simulink model "VB_RIFKF_UWB_INS25"  (R2023a)
settings: Solver=FixedStepAuto  StartTime=0.0  StopTime=500  FixedStep=0.01  RelTol=1e-3
InitFcn:
  | resilient_initNavigation1216;
  | init_param;
  | param_bias;
undefined symbols (not defined in the file or in its folder): dt, g0, gam0_rad, ISUS_flag, lp_GPS_sample_time, lp_Lidar_knoise, lp_Lidar_max, lp_Lidar_min, lp_Lidar_sample_time, lp_Lidar_seed, lp_UWB_knoise, lp_UWB_sample_time, lp_UWB_seed, lp_UWB_XY_max, lp_UWB_XY_min, magnitude, p, P0, P0_RIEKF, param, pd0, pe0, phi0_rad, pn0, psi, psi0_rad, state_dim, vd0, ve0, vn0
libraries: simulink_extras x108, simulink x89, dspstat3 x74, sharedtransform x61, matrix_library x11, sharedTrackingLibrary x8, aerolibconvert2 x5, aerolibtransform2 x5, dspfactors x3
(part 15 of 29)

== system VB_RIFKF_UWB_INS25/ISUS_RIEKF3/INS propogation3/att update ==
  dtheta : Inport
  gyro : Inport  Port=2
  quat_0 : Inport  Port=3  PortDimensions=4
  init_flag : Inport  Port=4
  Bus Creator1 : BusCreator  Inputs=1
  Constant : Constant  Value=dt
  Delay1 : Delay  DelayLength=1  InitialConditionSource=Input port  InitialCondition=0  ExternalReset=Level hold
      settings: InputPortMap=u0,r5,p4
  Detect Increase : simulink/Logic and Bit Operations/Detect Increase  vinit=0.0  OutDataTypeStr=boolean
  MATLAB Function : MATLAB Function  TreatAsAtomicUnit=on
  MATLAB Function2 : MATLAB Function  TreatAsAtomicUnit=on
  Quaternions to Direction Cosine Matrix : sharedtransform/Quaternions to  Direction Cosine Matrix  aMode=aMode
      settings: LibrarySourceBlock=|
      | aerolibtransform2/Quaternions to
      | Direction Cosine Matrix
  Scope : Scope
  Transpose : Math  Operator=transpose
  att_update1 : Outport
  wires:
  init_flag/1 -> Detect Increase/1
  quat_0/1 -> Quaternions to Direction Cosine Matrix/1
  gyro/1 -> MATLAB Function/2(w)  "w"
  Constant/1 -> MATLAB Function/3(dt)
  Quaternions to Direction Cosine Matrix/1 -> Transpose/1
  Transpose/1 -> Delay1/3
  Delay1/1 -> MATLAB Function/1(Rbn_k_1)
  Detect Increase/1 -> Delay1/2
  Bus Creator1/1 -> Delay1/1, att_update1/1
  MATLAB Function/1(Rbn) -> MATLAB Function2/2(Rbn)  "DCM_b_n"
  MATLAB Function2/1(Rbn_correct) -> Bus Creator1/1  "DCM_b_n"
  dtheta/1 -> MATLAB Function2/1(delta), Scope/1

== system VB_RIFKF_UWB_INS25/ISUS_RIEKF3/INS propogation3/gyro bias compensation ==
  raw <gyro_B_rad/s_LPF> : Inport
  ddg : Inport  Port=2
  Measuemrnt Enable Flag : Inport  Port=3
  QGC_init : Inport  Port=4
  Add1 : Sum
  Data Type Conversion4 : DataTypeConversion  OutDataTypeStr=single  SaturateOnIntegerOverflow=off  RndMeth=Floor
  Scope1 : Scope
  error compensation : Subsystem
      settings: PortSchema="{\"entries\":[{\"content\":{\"sides\":[{\"content\":{\"connectorIds\":[\"In1\",\"In2\"]},\"type\":\"ConnectorPlacement.EquallySpacedRectSide\",\"uuid\":\"380e61a1-8124-48da-8c16-e78a4b6c30a9\"},{\"content\":{\"connectorIds\":[\"Out1\"],\"side\":\"RIGHT\"},\"type\":\"ConnectorPlacement.EquallySpacedRectSide\",\"uuid\":\"dacfd24e-67c3-4852-b5f7-795187362148\"},{\"content\":{\"side\":\"TOP\"},\"type\":\"ConnectorPlacement.EquallySpacedRectSide\",\"uuid\":\"56579dc4-3963-4476-a5d7-e0c30cfcd11c\"},{\"content\":{\"connectorIds\":[\"In3\"],\"side\":\"BOTTOM\"},\"type\":\"ConnectorPlacement.EquallySpacedRectSide\",\"uuid\":\"fc24e139-e918-40f2-99cc-0ca16c0a4a58\"}]},\"type\":\"ConnectorPlacement.EquallySpacedConnector\",\"uuid\":\"3ce5c04a-f8d2-476b-8ef1-0541292dfd95\"}],\"packageUris\":[\"http://schema.mathworks.com/mf0/Connector/R2020b\"],\"version\":\"1.0\"}"
  wb : Outport  PortDimensions=3
  dg : Outport  Port=2  PortDimensions=3
  wires:
  Data Type Conversion4/1 -> wb/1
  raw <gyro_B_rad/s_LPF>/1 -> Add1/1
  error compensation/1(dg) -> Add1/2, Scope1/1, dg/1
  Measuemrnt Enable Flag/1 -> error compensation/2(Enable)
  Add1/1 -> Data Type Conversion4/1
  QGC_init/1 -> error compensation/3(QGC_init)
  ddg/1 -> error compensation/1(ddg)

== system VB_RIFKF_UWB_INS25/ISUS_RIEKF3/INS propogation3/vel//pos update ==
  dtheta : Inport
  <DCM_b_n> : Inport  Port=2
  Ab : Inport  Port=3
  v0 : Inport  Port=4
  p0 : Inport  Port=5
  QGC_init : Inport  Port=6
  dp : Inport  Port=7
  dv : Inport  Port=8
  Kinematic Equation : Subsystem
  QGC_init1 : InportShadow  Port=6
  pos update : Subsystem
  vel update : Subsystem
  p_k : Outport  PortDimensions=3
  V : Outport  Port=2  PortDimensions=3
  wires:
  QGC_init1/1 -> pos update/4(QGC_init)
  pos update/1(p_k) -> p_k/1
  p0/1 -> pos update/5(p0)
  dp/1 -> pos update/3(dp)
  v0/1 -> vel update/5(v0)
  dv/1 -> vel update/4(KFState_dv)
  Kinematic Equation/1(An) -> vel update/3(An)
  QGC_init/1 -> vel update/2(QGC_init)
  Ab/1 -> Kinematic Equation/2(Ab)
  <DCM_b_n>/1 -> Kinematic Equation/1(Cbn)
  vel update/1(vel_k) -> V/1, pos update/2(vel_k)
  dtheta/1 -> pos update/1(dtheta), vel update/1(dtheta)

== system VB_RIFKF_UWB_INS25/ISUS_RIEKF3/Subsystem/ISIU ==
  xk_k_1 : Inport
  xk_k_2 : Inport  Port=2
  xk_k_3 : Inport  Port=3
  pk_k_1 : Inport  Port=4
  pk_k_2 : Inport  Port=5
  pk_k_3 : Inport  Port=6
  1222bk : MATLAB Function  Commented=on  TreatAsAtomicUnit=on
  1222bk02 : MATLAB Function  Commented=on  TreatAsAtomicUnit=on
  Constant : Constant  Value=3
  Constant1 : Constant  OutDataTypeStr=boolean
  Constant11 : Constant  Commented=on  Value=[0.9;0.05;0.05]  OutDataTypeStr=single
  Data Type Conversion : DataTypeConversion  OutDataTypeStr=single  SaturateOnIntegerOverflow=off  RndMeth=Floor
  Data Type Conversion1 : DataTypeConversion  Commented=on  OutDataTypeStr=single  SaturateOnIntegerOverflow=off  RndMeth=Floor
  Delay1 : Delay  Commented=on  DelayLength=1  InitialConditionSource=Input port
      settings: InputPortMap=u0,p4
  Delay4 : Delay  Commented=on  DelayLength=1  InitialConditionSource=Input port
      settings: InputPortMap=u0,p4
  Digital Clock1 : DigitalClock  SampleTime=0.01
  MATLAB Function : MATLAB Function  TreatAsAtomicUnit=on
  MATLAB Function3 : MATLAB Function  Commented=on  TreatAsAtomicUnit=on
  MATLAB Function4 : MATLAB Function  TreatAsAtomicUnit=on
  Scope : Scope
  xk_k : Outport
  pk_k : Outport  Port=2
  xk_k_o1 : Outport  Port=3
  xk_k_o2 : Outport  Port=4
  xk_k_o3 : Outport  Port=5
  pk_k_o1 : Outport  Port=6
  pk_k_o2 : Outport  Port=7
  pk_k_o3 : Outport  Port=8
  wires:
  MATLAB Function/8(P_cov_system) -> pk_k/1
  MATLAB Function/7(system_pos) -> xk_k/1
  MATLAB Function/6(object3_cov) -> pk_k_o3/1
  MATLAB Function/5(object3_pos) -> xk_k_o3/1
  MATLAB Function/4(object2_cov) -> pk_k_o2/1
  MATLAB Function/3(object2_pos) -> xk_k_o2/1
  MATLAB Function/2(object1_cov) -> pk_k_o1/1
  MATLAB Function/1(object1_pos) -> xk_k_o1/1
  Data Type Conversion/1 -> Delay4/1
  Constant11/1 -> Delay4/2
  Data Type Conversion1/1 -> Delay1/1
  Constant/1 -> MATLAB Function/9(N)
  xk_k_3/1 -> MATLAB Function/8(object3_correct_pos)
  xk_k_2/1 -> MATLAB Function/7(object2_correct_pos)
  xk_k_1/1 -> MATLAB Function/6(object1_correct_pos)
  pk_k_3/1 -> MATLAB Function/3(inform_object3_correct)
  pk_k_2/1 -> MATLAB Function/2(inform_object2_correct)
  pk_k_1/1 -> MATLAB Function/1(inform_object1_correct)
  Constant1/1 -> MATLAB Function/10(flag), MATLAB Function4/2(u)
  Digital Clock1/1 -> MATLAB Function4/1(t)

== system VB_RIFKF_UWB_INS25/ISUS_RIEKF3/Subsystem/Subsystem ==
  X_mixed_RIEKF_M1 : Inport
  Bus Creator : BusCreator  Inputs=5
  Bus Creator1 : BusCreator  Inputs=1
  Selector : Selector  InputPortWidth=15  IndexOptions=Index vector (dialog)  Indices=[1 2 3]  OutputSizes=1
  Selector1 : Selector  InputPortWidth=15  IndexOptions=Index vector (dialog)  Indices=[4 5 6]  OutputSizes=1
  Selector2 : Selector  InputPortWidth=15  IndexOptions=Index vector (dialog)  Indices=[7 8 9]  OutputSizes=1
  Selector3 : Selector  InputPortWidth=15  IndexOptions=Index vector (dialog)  Indices=[10 11 12]  OutputSizes=1
  Selector4 : Selector  InputPortWidth=15  IndexOptions=Index vector (dialog)  Indices=[13 14 15]  OutputSizes=1
  Out1 : Outport
  wires:
  Selector3/1 -> Bus Creator/4  "KFState_dg"
  Selector1/1 -> Bus Creator/2  "KFState_dv"
  Selector2/1 -> Bus Creator/3  "KFState_dp"
  Bus Creator/1 -> Bus Creator1/1  "delta_state"
  Selector4/1 -> Bus Creator/5  "KFState_da"
  X_mixed_RIEKF_M1/1 -> Selector4/1, Selector3/1, Selector2/1, Selector1/1, Selector/1
  Selector/1 -> Bus Creator/1  "KFState_dtheta"
  Bus Creator1/1 -> Out1/1

== system VB_RIFKF_UWB_INS25/ISUS_RIEKF3/Subsystem/Subsystem1 ==
  X_mixed_RIEKF_M1 : Inport
  Bus Creator : BusCreator  Inputs=5
  Bus Creator1 : BusCreator  Inputs=1
  Selector : Selector  InputPortWidth=15  IndexOptions=Index vector (dialog)  Indices=[1 2 3]  OutputSizes=1
  Selector1 : Selector  InputPortWidth=15  IndexOptions=Index vector (dialog)  Indices=[4 5 6]  OutputSizes=1
  Selector2 : Selector  InputPortWidth=15  IndexOptions=Index vector (dialog)  Indices=[7 8 9]  OutputSizes=1
  Selector3 : Selector  InputPortWidth=15  IndexOptions=Index vector (dialog)  Indices=[10 11 12]  OutputSizes=1
  Selector4 : Selector  InputPortWidth=15  IndexOptions=Index vector (dialog)  Indices=[13 14 15]  OutputSizes=1
  Out1 : Outport
  wires:
  Bus Creator1/1 -> Out1/1
  Selector/1 -> Bus Creator/1  "KFState_dtheta"
  X_mixed_RIEKF_M1/1 -> Selector/1, Selector1/1, Selector2/1, Selector3/1, Selector4/1
  Selector4/1 -> Bus Creator/5  "KFState_da"
  Bus Creator/1 -> Bus Creator1/1  "delta_state"
  Selector2/1 -> Bus Creator/3  "KFState_dp"
  Selector1/1 -> Bus Creator/2  "KFState_dv"
  Selector3/1 -> Bus Creator/4  "KFState_dg"

== system VB_RIFKF_UWB_INS25/ISUS_RIEKF3/Subsystem/Subsystem2 ==
  X_mixed_RIEKF_M1 : Inport
  Bus Creator : BusCreator  Inputs=5
  Bus Creator1 : BusCreator  Inputs=1
  Selector : Selector  InputPortWidth=15  IndexOptions=Index vector (dialog)  Indices=[1 2 3]  OutputSizes=1
  Selector1 : Selector  InputPortWidth=15  IndexOptions=Index vector (dialog)  Indices=[4 5 6]  OutputSizes=1
  Selector2 : Selector  InputPortWidth=15  IndexOptions=Index vector (dialog)  Indices=[7 8 9]  OutputSizes=1
  Selector3 : Selector  InputPortWidth=15  IndexOptions=Index vector (dialog)  Indices=[10 11 12]  OutputSizes=1
  Selector4 : Selector  InputPortWidth=15  IndexOptions=Index vector (dialog)  Indices=[13 14 15]  OutputSizes=1
  Out1 : Outport
  wires:
  Selector3/1 -> Bus Creator/4  "KFState_dg"
  Selector1/1 -> Bus Creator/2  "KFState_dv"
  Selector2/1 -> Bus Creator/3  "KFState_dp"
  Bus Creator/1 -> Bus Creator1/1  "delta_state"
  Selector4/1 -> Bus Creator/5  "KFState_da"
  X_mixed_RIEKF_M1/1 -> Selector4/1, Selector3/1, Selector2/1, Selector1/1, Selector/1
  Selector/1 -> Bus Creator/1  "KFState_dtheta"
  Bus Creator1/1 -> Out1/1

== system VB_RIFKF_UWB_INS25/ISUS_RIEKF3/Subsystem/Subsystem3 ==
  X_mixed_RIEKF_M1 : Inport
  Bus Creator : BusCreator  Inputs=5
  Bus Creator1 : BusCreator  Inputs=1
  Selector : Selector  InputPortWidth=15  IndexOptions=Index vector (dialog)  Indices=[1 2 3]  OutputSizes=1
  Selector1 : Selector  InputPortWidth=15  IndexOptions=Index vector (dialog)  Indices=[4 5 6]  OutputSizes=1
  Selector2 : Selector  InputPortWidth=15  IndexOptions=Index vector (dialog)  Indices=[7 8 9]  OutputSizes=1
  Selector3 : Selector  InputPortWidth=15  IndexOptions=Index vector (dialog)  Indices=[10 11 12]  OutputSizes=1
  Selector4 : Selector  InputPortWidth=15  IndexOptions=Index vector (dialog)  Indices=[13 14 15]  OutputSizes=1
  Out1 : Outport
  wires:
  Bus Creator1/1 -> Out1/1
  Selector/1 -> Bus Creator/1  "KFState_dtheta"
  X_mixed_RIEKF_M1/1 -> Selector/1, Selector1/1, Selector2/1, Selector3/1, Selector4/1
  Selector4/1 -> Bus Creator/5  "KFState_da"
  Bus Creator/1 -> Bus Creator1/1  "delta_state"
  Selector2/1 -> Bus Creator/3  "KFState_dp"
  Selector1/1 -> Bus Creator/2  "KFState_dv"
  Selector3/1 -> Bus Creator/4  "KFState_dg"

== system VB_RIFKF_UWB_INS25/No.1_Sensor_Data_Process/GPS_Data_Process/LLA2NED ==
  note: Vecef2ned
  gps_LLA_rad : Inport
  GPSfixtype : Inport  Port=2
  GPS_Vecef_m/s : Inport  Port=3
  QGC_sensor_reinit : Inport  Port=4
  Angle Conversion1 : aerolibconvert2/Angle Conversion  IU=deg  OU=rad
  Bus Creator : BusCreator  Inputs=3
  Bus Creator1 : BusCreator  Inputs=3
  Bus Creator2 : BusCreator  Inputs=3
  Bus Selector : BusSelector  OutputSignals=lon_gps,lat_gps
  Bus Selector1 : BusSelector  OutputSignals=lat_gps,lon_gps,H_gps
  Constant1 : Constant  Value=-90
  Constant4 : Constant  Value=0
  Data Type Conversion{,1..6} (7 alike) : DataTypeConversion  OutDataTypeStr=single  SaturateOnIntegerOverflow=off  RndMeth=Floor
  Demux{,1..3} (4 alike) : Demux  Outputs=3
  Detect Increase : simulink/Logic and Bit Operations/Detect Increase  vinit=0.0  OutDataTypeStr=boolean
  Digital Clock : DigitalClock  SampleTime=0.01
  Direction Cosine Matrix ECEF to NED : aerolibtransform2/Direction Cosine Matrix ECEF to NED  Commented=on
  Divide1 : Product  Inputs=**  Multiplication=Matrix(*)
  Gain : Gain  Gain=-1
  LLA to ECEF Position : LLA2ECEF  R=6378137
  LLA to ECEF Position1 : LLA2ECEF  R=6378137
  MATLAB Function2 : MATLAB Function  TreatAsAtomicUnit=on
  Mux2 : Mux  Inputs=3
  Mux5 : Mux  Inputs=2
  Mux6 : Mux  Inputs=2
  Product : Product  Commented=on  Multiplication=Matrix(*)
  Radians to Degrees{,1..3} (4 alike) : simulink_extras/Transformations/Radians to Degrees
  Radians to Degrees4 : simulink_extras/Transformations/Radians to Degrees  Commented=on
  Rotation Angles to Direction Cosine Matrix : sharedtransform/Rotation Angles to Direction Cosine Matrix  rotationOrder=ZYX  aMode=aMode
  Scope : Scope  NumInputPorts=2
  Scope1 : Scope
  Scope2 : Scope  NumInputPorts=2
  Selector2 : Selector  Commented=on  InputPortWidth=3  IndexOptions=Index vector (dialog)  Indices=[1 2]  OutputSizes=1
  Sum : Sum  Inputs=|++
  Sum1 : Sum  Inputs=|+-
  initGPSLLA : MATLAB Function  TreatAsAtomicUnit=on
  "gpsposNEDout " : Outport
  gpsvNEDout : Outport  Port=2
  GPS0 : Outport  Port=3
  gpsposNED_noerr : Outport  Port=4
  wires:
  initGPSLLA/2(init_GPSLLAflag) -> Scope/1
  initGPSLLA/1(gpsLLA0_rad) -> Scope/2, Demux/1
  Detect Increase/1 -> initGPSLLA/1(QGCinitflag)
  Data Type Conversion3/1 -> gpsvNEDout/1  "gpspos_N"
  Radians to Degrees4/1 -> Direction Cosine Matrix ECEF to NED/1
  Selector2/1 -> Radians to Degrees4/1
  Direction Cosine Matrix ECEF to NED/1 -> Product/1
  GPS_Vecef_m/s/1 -> Product/2, Data Type Conversion3/1
  Radians to Degrees3/1 -> Mux5/2
  Radians to Degrees2/1 -> Mux5/1
  Angle Conversion1/1 -> Sum/2
  Data Type Conversion2/1 -> Bus Creator1/3  "gpspos_D"
  Data Type Conversion1/1 -> Bus Creator1/2  "gpspos_E"
  Data Type Conversion/1 -> Bus Creator1/1  "gpspos_N"
  QGC_sensor_reinit/1 -> Detect Increase/1
  Radians to Degrees1/1 -> Mux6/2
  Radians to Degrees/1 -> Mux6/1
  gps_LLA_rad/1 -> Demux1/1, Selector2/1, initGPSLLA/3(gps_LLA_rad)
  Bus Selector1/3 -> LLA to ECEF Position/2  "<H_gps>"
  Bus Selector1/2 -> Radians to Degrees3/1  "<lon_gps>"
  Bus Selector1/1 -> Radians to Degrees2/1  "<lat_gps>"
  Bus Selector/1 -> Mux2/1  "<lon_gps>"
  Bus Selector/2 -> Gain/1  "<lat_gps>"
  Sum/1 -> Mux2/2
  Demux1/2 -> Radians to Degrees1/1
  LLA to ECEF Position/1 -> Sum1/2
  Constant1/1 -> Angle Conversion1/1
  Rotation Angles to Direction Cosine Matrix/1 -> Divide1/1
  Mux2/1 -> Rotation Angles to Direction Cosine Matrix/1
  Demux1/1 -> Radians to Degrees/1
  Sum1/1 -> Divide1/2
  Constant4/1 -> Mux2/3
  LLA to ECEF Position1/1 -> Sum1/1
  Gain/1 -> Sum/1
  Mux5/1 -> LLA to ECEF Position/1
  Mux6/1 -> LLA to ECEF Position1/1
  Demux1/3 -> LLA to ECEF Position1/2
  Demux/1 -> Bus Creator/1  "lat_gps"
  Demux/2 -> Bus Creator/2  "lon_gps"
  Demux/3 -> Bus Creator/3  "H_gps"
  Bus Creator/1 -> GPS0/1, Bus Selector1/1, Bus Selector/1
  Demux3/1 -> Data Type Conversion/1  "gpspos_N"
  Demux3/2 -> Data Type Conversion1/1  "gpspos_E"
  Demux3/3 -> Data Type Conversion2/1  "gpspos_D"
  Bus Creator1/1 -> Scope1/1, "gpsposNEDout "/1
  GPSfixtype/1 -> initGPSLLA/2(GPSfixtype)
  Digital Clock/1 -> MATLAB Function2/1(t)
  Bus Creator2/1 -> gpsposNED_noerr/1
  Demux2/3 -> Data Type Conversion6/1  "gpspos_D"
  Demux2/2 -> Data Type Conversion5/1  "gpspos_E"
  Demux2/1 -> Data Type Conversion4/1  "gpspos_N"
  Data Type Conversion4/1 -> Bus Creator2/1  "gpspos_N"
  Data Type Conversion5/1 -> Bus Creator2/2  "gpspos_E"
  Data Type Conversion6/1 -> Bus Creator2/3  "gpspos_D"
  Divide1/1 -> Demux3/1, Scope2/1, Demux2/1, Scope2/2, MATLAB Function2/2(u)

== system VB_RIFKF_UWB_INS25/No.1_Sensor_Data_Process/GPS_Data_Process/heading_GPS ==
  Vned : Inport
  Atan2 : Trigonometry  Operator=atan2
  Compare To Constant : simulink/Logic and Bit Operations/Compare To Constant  relop=>=  const=0.8  OutDataTypeStr=boolean
  Math Function : Math  Operator=magnitude^2  SignedPower=on
  Moving Average1 : dspstat3/Moving Average  Commented=on  Method=Sliding window  ForgettingFactorPort=off  SpecifyWindowLength=on  WindowLength=10  OverlapLength=9  AllowArbitraryInputLength=off  ForgettingFactor=0.9  SimulateUsing=Code generation
  Scope : Scope  NumInputPorts=2
  Scope1 : Scope
  Selector2 : Selector  InputPortWidth=3  IndexOptions=Index vector (dialog)  Indices=[2]  OutputSizes=1
  Selector3 : Selector  InputPortWidth=3  IndexOptions=Index vector (dialog)  Indices=[1]  OutputSizes=1
  Selector4 : Selector  InputPortWidth=3  IndexOptions=Index vector (dialog)  Indices=[1 2]  OutputSizes=1
  Sqrt : Sqrt
  Sum of Elements : Sum  Inputs=+
  heading_GPS_rad : Outport
  heading_GPS_valid : Outport  Port=2
  wires:
  Atan2/1 -> heading_GPS_rad/1, Scope/2, Scope/1
  Compare To Constant/1 -> heading_GPS_valid/1, Scope1/1
  Sqrt/1 -> Compare To Constant/1
  Selector4/1 -> Math Function/1
  Sum of Elements/1 -> Sqrt/1
  Selector3/1 -> Atan2/2
  Vned/1 -> Selector3/1, Selector4/1, Selector2/1
  Math Function/1 -> Sum of Elements/1
  Selector2/1 -> Atan2/1

== system VB_RIFKF_UWB_INS25/No.1_Sensor_Data_Process/IMU_Data_Process/Bias Eliminate ==
  gyro_B_rad/s_ori : Inport
  Data Type Conversion : DataTypeConversion  OutDataTypeStr=single  SaturateOnIntegerOverflow=off  RndMeth=Floor
  Digital Clock : DigitalClock
  Memory : Memory
  Scope : Scope
  Subsystem : Subsystem
  Sum : Sum  Inputs=|+-
  Switch : Switch  Criteria=u2 > Threshold  Threshold=5  SaturateOnIntegerOverflow=off  InputSameDT=off
  Out1 : Outport
  wires:
  Memory/1 -> Switch/1
  Switch/1 -> Memory/1, Scope/1
  Subsystem/1(mean_data) -> Switch/3
  Digital Clock/1 -> Switch/2
  Sum/1 -> Data Type Conversion/1
  gyro_B_rad/s_ori/1 -> Sum/1, Subsystem/1(data)
  Data Type Conversion/1 -> Out1/1

== system VB_RIFKF_UWB_INS25/No.1_Sensor_Data_Process/IMU_Data_Process/accl_preprocessing2 ==
  note: front-right-dowm
  accl_B_m/s_ori : Inport
  Constant2 : Constant  Value=1/dt  OutDataTypeStr=single
  Constant4 : Constant  Value=1/dt  OutDataTypeStr=single
  Constant6 : Constant  Value=1/dt  OutDataTypeStr=single
  Constant7 : Constant  Value=param.proces.imu_gyro_cutoff_freq  OutDataTypeStr=single
  Demux : Demux  Outputs=3
  MATLAB Function1 : MATLAB Function  TreatAsAtomicUnit=on
  MATLAB Function2 : MATLAB Function  TreatAsAtomicUnit=on
  MATLAB Function3 : MATLAB Function  TreatAsAtomicUnit=on
  Vector Concatenate : Concatenate  NumInputs=3
  accl_B_m/s2_LPF : Outport
  wires:
  MATLAB Function2/1(curr_output) -> Vector Concatenate/1  "wx"
  MATLAB Function1/1(curr_output) -> Vector Concatenate/2  "wy"
  MATLAB Function3/1(curr_output) -> Vector Concatenate/3  "wz"
  Constant7/1 -> MATLAB Function1/3(cutoff_freq), MATLAB Function3/3(cutoff_freq), MATLAB Function2/3(cutoff_freq)
  Demux/3 -> MATLAB Function3/1(curr_input)
  Constant6/1 -> MATLAB Function3/2(sample_freq)
  Demux/2 -> MATLAB Function1/1(curr_input)
  Demux/1 -> MATLAB Function2/1(curr_input)
  accl_B_m/s_ori/1 -> Demux/1
  Constant2/1 -> MATLAB Function1/2(sample_freq)
  Constant4/1 -> MATLAB Function2/2(sample_freq)
  Vector Concatenate/1 -> accl_B_m/s2_LPF/1

== system VB_RIFKF_UWB_INS25/No.1_Sensor_Data_Process/IMU_Data_Process/gyro_preprocessing2 ==
  note: rad/s
  note: front-right-dowm
  gyro_B_rad/s_ori : Inport
  Constant2 : Constant  Value=1/dt  OutDataTypeStr=single
  Constant4 : Constant  Value=1/dt  OutDataTypeStr=single
  Constant6 : Constant  Value=1/dt  OutDataTypeStr=single
  Constant7 : Constant  Value=param.proces.imu_gyro_cutoff_freq  OutDataTypeStr=single
  Demux : Demux  Outputs=3
  MATLAB Function1 : MATLAB Function  TreatAsAtomicUnit=on
  MATLAB Function2 : MATLAB Function  TreatAsAtomicUnit=on
  MATLAB Function3 : MATLAB Function  TreatAsAtomicUnit=on
  Scope : Scope  NumInputPorts=2
  Vector Concatenate : Concatenate  NumInputs=3
  gyro_B_rad/s_LPF : Outport  PortDimensions=3
  wires:
  Vector Concatenate/1 -> gyro_B_rad/s_LPF/1
  Constant4/1 -> MATLAB Function2/2(sample_freq)
  Constant2/1 -> MATLAB Function1/2(sample_freq)
  gyro_B_rad/s_ori/1 -> Demux/1
  Demux/1 -> Scope/2, MATLAB Function2/1(curr_input)
  Demux/2 -> MATLAB Function1/1(curr_input)
  Constant6/1 -> MATLAB Function3/2(sample_freq)
  Demux/3 -> MATLAB Function3/1(curr_input)
  Constant7/1 -> MATLAB Function2/3(cutoff_freq), MATLAB Function1/3(cutoff_freq), MATLAB Function3/3(cutoff_freq)
  MATLAB Function3/1(curr_output) -> Vector Concatenate/3  "wz"
  MATLAB Function1/1(curr_output) -> Vector Concatenate/2  "wy"
  MATLAB Function2/1(curr_output) -> Vector Concatenate/1  "wx"

== system VB_RIFKF_UWB_INS25/No.1_Sensor_Data_Process/Magn_Data_Process/Magn_preprocessing ==
  note: front-right-dowm
  Magn_B_rad/s_ori : Inport
  Constant2 : Constant  Value=1/dt  OutDataTypeStr=single
  Constant4 : Constant  Value=1/dt  OutDataTypeStr=single
  Constant6 : Constant  Value=1/dt  OutDataTypeStr=single
  Constant7 : Constant  Value=param.proces.imu_gyro_cutoff_freq  OutDataTypeStr=single
  Demux : Demux  Outputs=3
  MATLAB Function1 : MATLAB Function  TreatAsAtomicUnit=on
  MATLAB Function2 : MATLAB Function  TreatAsAtomicUnit=on
  MATLAB Function3 : MATLAB Function  TreatAsAtomicUnit=on
  Scope : Scope  NumInputPorts=2
  Vector Concatenate : Concatenate  NumInputs=3
  Magn_B_rad/s_LPF : Outport
  wires:
  MATLAB Function2/1(curr_output) -> Vector Concatenate/1  "wx"
  MATLAB Function1/1(curr_output) -> Vector Concatenate/2  "wy"
  MATLAB Function3/1(curr_output) -> Vector Concatenate/3  "wz"
  Constant7/1 -> MATLAB Function3/3(cutoff_freq), MATLAB Function1/3(cutoff_freq), MATLAB Function2/3(cutoff_freq)
  Demux/3 -> MATLAB Function3/1(curr_input)
  Constant6/1 -> MATLAB Function3/2(sample_freq)
  Demux/2 -> MATLAB Function1/1(curr_input)
  Demux/1 -> MATLAB Function2/1(curr_input), Scope/2
  Magn_B_rad/s_ori/1 -> Demux/1
  Constant2/1 -> MATLAB Function1/2(sample_freq)
  Constant4/1 -> MATLAB Function2/2(sample_freq)
  Vector Concatenate/1 -> Magn_B_rad/s_LPF/1

== system VB_RIFKF_UWB_INS25/No.1_Sensor_Data_Process/Subsystem/TD_baro ==
  H_baro : Inport
  Constant1 : Constant  Value=dt  OutDataTypeStr=single
  Constant3 : Constant  Value=0.1  OutDataTypeStr=single
  Constant4 : Constant  Value=900  OutDataTypeStr=single
  Delay1 : Delay  DelayLength=1  InitialConditionSource=Input port
      settings: InputPortMap=u0,p4
  MATLAB Function2 : MATLAB Function  TreatAsAtomicUnit=on
  Memory : Memory  InheritSampleTime=on
  Scope : Scope  NumInputPorts=3
  vH_baro_TD : Outport
  H_baro_TD : Outport  Port=2
  wires:
  MATLAB Function2/2(u2) -> Memory/1
  MATLAB Function2/1(u1) -> Delay1/1
  Constant4/1 -> MATLAB Function2/6(r)
  Constant1/1 -> MATLAB Function2/1(T)
  Constant3/1 -> MATLAB Function2/5(h)
  Memory/1 -> Scope/2, vH_baro_TD/1, MATLAB Function2/4("u2 ")
  H_baro/1 -> Scope/1, MATLAB Function2/2(u0), Delay1/2
  Delay1/1 -> MATLAB Function2/3("u1 "), Scope/3, H_baro_TD/1

== system VB_RIFKF_UWB_INS25/No.1_Sensor_Data_Process/TOF_Data_Process/TD_baro ==
  H_TOF : Inport
  Constant1 : Constant  Value=dt  OutDataTypeStr=single
  Constant3 : Constant  Value=0.04  OutDataTypeStr=single
  Constant4 : Constant  Value=600  OutDataTypeStr=single
  Delay1 : Delay  DelayLength=1  InitialConditionSource=Input port
      settings: InputPortMap=u0,p4
  MATLAB Function2 : MATLAB Function  TreatAsAtomicUnit=on
  Memory : Memory  InheritSampleTime=on
  Scope : Scope  NumInputPorts=3
  vH_TOF_TD : Outport
  H_TOF_TD : Outport  Port=2
  wires:
  MATLAB Function2/2(u2) -> Memory/1
  MATLAB Function2/1(u1) -> Delay1/1
  Constant4/1 -> MATLAB Function2/6(r)
  Constant1/1 -> MATLAB Function2/1(T)
  Constant3/1 -> MATLAB Function2/5(h)
  Memory/1 -> Scope/2, vH_TOF_TD/1, MATLAB Function2/4("u2 ")
  H_TOF/1 -> Scope/1, MATLAB Function2/2(u0), Delay1/2
  Delay1/1 -> MATLAB Function2/3("u1 "), Scope/3, H_TOF_TD/1

== system VB_RIFKF_UWB_INS25/No.1_Sensor_Data_Process/TOF_Data_Process/reinit_TOF ==
  QGC_sensor_reinit : Inport
  Data : Inport  Port=2
  Detect Increase : simulink/Logic and Bit Operations/Detect Increase  vinit=0.0  OutDataTypeStr=boolean
  Switch : Switch  Criteria=u2 > Threshold  SaturateOnIntegerOverflow=off  InputSameDT=off
  Unit Delay : UnitDelay  SampleTime=-1  HasFrameUpgradeWarning=on
  dataout : Outport
  wires:
  QGC_sensor_reinit/1 -> Detect Increase/1
  Detect Increase/1 -> Switch/2
  Switch/1 -> Unit Delay/1, dataout/1
  Data/1 -> Switch/1
  Unit Delay/1 -> Switch/3

== system VB_RIFKF_UWB_INS25/No.1_Sensor_Data_Process/baro_Data_Process/Pressure2Height ==
  baro : Inport
  Add : Sum  Inputs=+-
  Constant : Constant  OutDataTypeStr=single
  Constant1 : Constant  Value=1/5.255  OutDataTypeStr=single
  Gain : Gain  Gain=1/1.01325
  Gain1 : Gain  Gain=44330
  Math Function : Math  Operator=pow  SignedPower=on
  H_baro : Outport
  wires:
  baro/1 -> Gain/1
  Gain1/1 -> H_baro/1
  Add/1 -> Gain1/1
  Constant/1 -> Add/1
  Math Function/1 -> Add/2
  Constant1/1 -> Math Function/2
  Gain/1 -> Math Function/1

== system VB_RIFKF_UWB_INS25/No.1_Sensor_Data_Process/baro_Data_Process/TD_baro ==
  H_baro : Inport
  Constant1 : Constant  Value=dt  OutDataTypeStr=single
  Constant3 : Constant  Value=0.23  OutDataTypeStr=single
  Constant4 : Constant  Value=900  OutDataTypeStr=single
  Delay1 : Delay  DelayLength=1  InitialConditionSource=Input port
      settings: InputPortMap=u0,p4
  MATLAB Function2 : MATLAB Function  TreatAsAtomicUnit=on
  Memory : Memory  InheritSampleTime=on
  Scope : Scope  NumInputPorts=3
  vH_baro_TD : Outport
  H_baro_TD : Outport  Port=2
  wires:
  MATLAB Function2/2(u2) -> Memory/1
  MATLAB Function2/1(u1) -> Delay1/1
  Constant4/1 -> MATLAB Function2/6(r)
  Constant1/1 -> MATLAB Function2/1(T)
  Constant3/1 -> MATLAB Function2/5(h)
  Memory/1 -> Scope/2, vH_baro_TD/1, MATLAB Function2/4("u2 ")
  H_baro/1 -> Scope/1, MATLAB Function2/2(u0), Delay1/2
  Delay1/1 -> MATLAB Function2/3("u1 "), Scope/3, H_baro_TD/1

== system VB_RIFKF_UWB_INS25/No.1_Sensor_Data_Process/baro_Data_Process/TemCompensate1 ==
  baro_tem : Inport
  Add : Sum  Inputs=+++
  Constant2 : Constant  Value=-1663  OutDataTypeStr=single
  Gain : Gain  Gain=-1.6
  Gain1 : Gain  Gain=102.5
  Product : Product
  bias : Outport
  wires:
  baro_tem/1 -> Gain1/1, Product/2, Product/1
  Constant2/1 -> Add/3
  Product/1 -> Gain/1
  Gain/1 -> Add/1
  Add/1 -> bias/1
  Gain1/1 -> Add/2

== system VB_RIFKF_UWB_INS25/No.1_Sensor_Data_Process/baro_Data_Process/reinit_baro0 ==
  QGC_sensor_reinit : Inport
  Data : Inport  Port=2
  Detect Increase : simulink/Logic and Bit Operations/Detect Increase  vinit=0.0  OutDataTypeStr=boolean
  Switch : Switch  Criteria=u2 > Threshold  SaturateOnIntegerOverflow=off  InputSameDT=off
  Unit Delay : UnitDelay  SampleTime=-1  HasFrameUpgradeWarning=on
  dataout : Outport
  wires:
  QGC_sensor_reinit/1 -> Detect Increase/1
  Detect Increase/1 -> Switch/2
  Switch/1 -> Unit Delay/1, dataout/1
  Data/1 -> Switch/1
  Unit Delay/1 -> Switch/3

== system VB_RIFKF_UWB_INS25/No.1_Sensor_Data_Process/baro_Data_Process/reinit_baro1 ==
  QGC_sensor_reinit : Inport
  Data : Inport  Port=2
  Detect Increase : simulink/Logic and Bit Operations/Detect Increase  vinit=0.0  OutDataTypeStr=boolean
  Switch : Switch  Criteria=u2 > Threshold  SaturateOnIntegerOverflow=off  InputSameDT=off
  Unit Delay : UnitDelay  SampleTime=-1  HasFrameUpgradeWarning=on
  dataout : Outport
  wires:
  Unit Delay/1 -> Switch/3
  Data/1 -> Switch/1
  Switch/1 -> dataout/1, Unit Delay/1
  Detect Increase/1 -> Switch/2
  QGC_sensor_reinit/1 -> Detect Increase/1

== system VB_RIFKF_UWB_INS25/No.1_Sensor_Data_Process1/GPS_Data_Process/LLA2NED ==
  note: Vecef2ned
  gps_LLA_rad : Inport
  GPSfixtype : Inport  Port=2
  GPS_Vecef_m/s : Inport  Port=3
  QGC_sensor_reinit : Inport  Port=4
  GPS0 : Inport  Port=5
  Angle Conversion1 : aerolibconvert2/Angle Conversion  IU=deg  OU=rad
  Bus Creator : BusCreator  Inputs=3
  Bus Creator1 : BusCreator  Inputs=3
  Bus Selector : BusSelector  OutputSignals=lon_gps,lat_gps
  Bus Selector1 : BusSelector  OutputSignals=lat_gps,lon_gps,H_gps
  Constant1 : Constant  Value=-90
  Constant4 : Constant  Value=0
  Data Type Conversion{,1..3} (4 alike) : DataTypeConversion  OutDataTypeStr=single  SaturateOnIntegerOverflow=off  RndMeth=Floor
  Demux : Demux  Outputs=3
  Demux1 : Demux  Outputs=3
  Demux3 : Demux  Outputs=3
  Detect Increase : simulink/Logic and Bit Operations/Detect Increase  vinit=0.0  OutDataTypeStr=boolean
  Digital Clock : DigitalClock  SampleTime=0.01
  Direction Cosine Matrix ECEF to NED : aerolibtransform2/Direction Cosine Matrix ECEF to NED  Commented=on
  Divide1 : Product  Inputs=**  Multiplication=Matrix(*)
  Gain : Gain  Gain=-1
  LLA to ECEF Position : LLA2ECEF  R=6378137
  LLA to ECEF Position1 : LLA2ECEF  R=6378137
  MATLAB Function2 : MATLAB Function  TreatAsAtomicUnit=on
  Mux2 : Mux  Inputs=3
  Mux5 : Mux  Inputs=2
  Mux6 : Mux  Inputs=2
  Product : Product  Commented=on  Multiplication=Matrix(*)
  Radians to Degrees{,1..3} (4 alike) : simulink_extras/Transformations/Radians to Degrees
  Radians to Degrees4 : simulink_extras/Transformations/Radians to Degrees  Commented=on
  Rotation Angles to Direction Cosine Matrix : sharedtransform/Rotation Angles to Direction Cosine Matrix  rotationOrder=ZYX  aMode=aMode
  Scope1 : Scope
  Selector2 : Selector  Commented=on  InputPortWidth=3  IndexOptions=Index vector (dialog)  Indices=[1 2]  OutputSizes=1
  Sum : Sum  Inputs=|++
  Sum1 : Sum  Inputs=|+-
  initGPSLLA : MATLAB Function  TreatAsAtomicUnit=on
  "gpsposNEDout " : Outport
  gpsvNEDout : Outport  Port=2
  wires:
  GPSfixtype/1 -> initGPSLLA/2(GPSfixtype)
  Bus Creator1/1 -> "gpsposNEDout "/1, Scope1/1
  Demux3/3 -> Data Type Conversion2/1  "gpspos_D"
  Demux3/2 -> Data Type Conversion1/1  "gpspos_E"
  Demux3/1 -> Data Type Conversion/1  "gpspos_N"
  Bus Creator/1 -> Bus Selector/1, Bus Selector1/1
  Demux/3 -> Bus Creator/3  "H_gps"
  Demux/2 -> Bus Creator/2  "lon_gps"
  Demux/1 -> Bus Creator/1  "lat_gps"
  Demux1/3 -> LLA to ECEF Position1/2
  Mux6/1 -> LLA to ECEF Position1/1
  Mux5/1 -> LLA to ECEF Position/1
  Gain/1 -> Sum/1
  LLA to ECEF Position1/1 -> Sum1/1
  Constant4/1 -> Mux2/3
  Sum1/1 -> Divide1/2
  Demux1/1 -> Radians to Degrees/1
  Mux2/1 -> Rotation Angles to Direction Cosine Matrix/1
  Rotation Angles to Direction Cosine Matrix/1 -> Divide1/1
  Constant1/1 -> Angle Conversion1/1
  LLA to ECEF Position/1 -> Sum1/2
  Demux1/2 -> Radians to Degrees1/1
  Sum/1 -> Mux2/2
  Bus Selector/2 -> Gain/1  "<lat_gps>"
  Bus Selector/1 -> Mux2/1  "<lon_gps>"
  Bus Selector1/1 -> Radians to Degrees2/1  "<lat_gps>"
  Bus Selector1/2 -> Radians to Degrees3/1  "<lon_gps>"
  Bus Selector1/3 -> LLA to ECEF Position/2  "<H_gps>"
  gps_LLA_rad/1 -> initGPSLLA/3(gps_LLA_rad), Selector2/1, Demux1/1
  Radians to Degrees/1 -> Mux6/1
  Radians to Degrees1/1 -> Mux6/2
  QGC_sensor_reinit/1 -> Detect Increase/1
  Data Type Conversion/1 -> Bus Creator1/1  "gpspos_N"
  Data Type Conversion1/1 -> Bus Creator1/2  "gpspos_E"
  Data Type Conversion2/1 -> Bus Creator1/3  "gpspos_D"
  Angle Conversion1/1 -> Sum/2
  Radians to Degrees2/1 -> Mux5/1
  Radians to Degrees3/1 -> Mux5/2
  GPS_Vecef_m/s/1 -> Data Type Conversion3/1, Product/2
  Direction Cosine Matrix ECEF to NED/1 -> Product/1
  Selector2/1 -> Radians to Degrees4/1
  Radians to Degrees4/1 -> Direction Cosine Matrix ECEF to NED/1
  Data Type Conversion3/1 -> gpsvNEDout/1  "gpspos_N"
  Detect Increase/1 -> initGPSLLA/1(QGCinitflag)
  initGPSLLA/1(gpsLLA0_rad) -> Demux/1
  Divide1/1 -> Demux3/1, MATLAB Function2/2(u)
  Digital Clock/1 -> MATLAB Function2/1(t)

== system VB_RIFKF_UWB_INS25/No.1_Sensor_Data_Process1/GPS_Data_Process/heading_GPS ==
  Vned : Inport
  Atan2 : Trigonometry  Operator=atan2
  Compare To Constant : simulink/Logic and Bit Operations/Compare To Constant  relop=>=  const=0.8  OutDataTypeStr=boolean
  Math Function : Math  Operator=magnitude^2  SignedPower=on
  Moving Average1 : dspstat3/Moving Average  Commented=on  Method=Sliding window  ForgettingFactorPort=off  SpecifyWindowLength=on  WindowLength=10  OverlapLength=9  AllowArbitraryInputLength=off  ForgettingFactor=0.9  SimulateUsing=Code generation
  Scope : Scope  NumInputPorts=2
  Scope1 : Scope
  Selector2 : Selector  InputPortWidth=3  IndexOptions=Index vector (dialog)  Indices=[2]  OutputSizes=1
  Selector3 : Selector  InputPortWidth=3  IndexOptions=Index vector (dialog)  Indices=[1]  OutputSizes=1
  Selector4 : Selector  InputPortWidth=3  IndexOptions=Index vector (dialog)  Indices=[1 2]  OutputSizes=1
  Sqrt : Sqrt
  Sum of Elements : Sum  Inputs=+
  heading_GPS_rad : Outport
  heading_GPS_valid : Outport  Port=2
  wires:
  Selector2/1 -> Atan2/1
  Math Function/1 -> Sum of Elements/1
  Vned/1 -> Selector2/1, Selector4/1, Selector3/1
  Selector3/1 -> Atan2/2
  Sum of Elements/1 -> Sqrt/1
  Selector4/1 -> Math Function/1
  Sqrt/1 -> Compare To Constant/1
  Compare To Constant/1 -> Scope1/1, heading_GPS_valid/1
  Atan2/1 -> Scope/1, Scope/2, heading_GPS_rad/1

== system VB_RIFKF_UWB_INS25/No.1_Sensor_Data_Process1/IMU_Data_Process/Bias Eliminate ==
  gyro_B_rad/s_ori : Inport
  Data Type Conversion : DataTypeConversion  OutDataTypeStr=single  SaturateOnIntegerOverflow=off  RndMeth=Floor
  Digital Clock : DigitalClock
  Memory : Memory
  Scope : Scope
  Subsystem : Subsystem
  Sum : Sum  Inputs=|+-
  Switch : Switch  Criteria=u2 > Threshold  Threshold=5  SaturateOnIntegerOverflow=off  InputSameDT=off
  Out1 : Outport
  wires:
  Data Type Conversion/1 -> Out1/1
  gyro_B_rad/s_ori/1 -> Subsystem/1(data), Sum/1
  Sum/1 -> Data Type Conversion/1
  Digital Clock/1 -> Switch/2
  Subsystem/1(mean_data) -> Switch/3
  Switch/1 -> Scope/1, Memory/1
  Memory/1 -> Switch/1

== system VB_RIFKF_UWB_INS25/No.1_Sensor_Data_Process1/IMU_Data_Process/accl_preprocessing2 ==
  note: front-right-dowm
  accl_B_m/s_ori : Inport
  Constant2 : Constant  Value=1/dt  OutDataTypeStr=single
  Constant4 : Constant  Value=1/dt  OutDataTypeStr=single
  Constant6 : Constant  Value=1/dt  OutDataTypeStr=single
  Constant7 : Constant  Value=param.proces.imu_gyro_cutoff_freq  OutDataTypeStr=single
  Demux : Demux  Outputs=3
  MATLAB Function1 : MATLAB Function  TreatAsAtomicUnit=on
  MATLAB Function2 : MATLAB Function  TreatAsAtomicUnit=on
  MATLAB Function3 : MATLAB Function  TreatAsAtomicUnit=on
  Vector Concatenate : Concatenate  NumInputs=3
  accl_B_m/s2_LPF : Outport
  wires:
  Vector Concatenate/1 -> accl_B_m/s2_LPF/1
  Constant4/1 -> MATLAB Function2/2(sample_freq)
  Constant2/1 -> MATLAB Function1/2(sample_freq)
  accl_B_m/s_ori/1 -> Demux/1
  Demux/1 -> MATLAB Function2/1(curr_input)
  Demux/2 -> MATLAB Function1/1(curr_input)
  Constant6/1 -> MATLAB Function3/2(sample_freq)
  Demux/3 -> MATLAB Function3/1(curr_input)
  Constant7/1 -> MATLAB Function2/3(cutoff_freq), MATLAB Function3/3(cutoff_freq), MATLAB Function1/3(cutoff_freq)
  MATLAB Function3/1(curr_output) -> Vector Concatenate/3  "wz"
  MATLAB Function1/1(curr_output) -> Vector Concatenate/2  "wy"
  MATLAB Function2/1(curr_output) -> Vector Concatenate/1  "wx"

== system VB_RIFKF_UWB_INS25/No.1_Sensor_Data_Process1/IMU_Data_Process/gyro_preprocessing2 ==
  note: front-right-dowm
  note: rad/s
  gyro_B_rad/s_ori : Inport
  Constant2 : Constant  Value=1/dt  OutDataTypeStr=single
  Constant4 : Constant  Value=1/dt  OutDataTypeStr=single
  Constant6 : Constant  Value=1/dt  OutDataTypeStr=single
  Constant7 : Constant  Value=param.proces.imu_gyro_cutoff_freq  OutDataTypeStr=single
  Demux : Demux  Outputs=3
  MATLAB Function1 : MATLAB Function  TreatAsAtomicUnit=on
  MATLAB Function2 : MATLAB Function  TreatAsAtomicUnit=on
  MATLAB Function3 : MATLAB Function  TreatAsAtomicUnit=on
  Scope : Scope  NumInputPorts=2
  Vector Concatenate : Concatenate  NumInputs=3
  gyro_B_rad/s_LPF : Outport  PortDimensions=3
  wires:
  MATLAB Function2/1(curr_output) -> Vector Concatenate/1  "wx"
  MATLAB Function1/1(curr_output) -> Vector Concatenate/2  "wy"
  MATLAB Function3/1(curr_output) -> Vector Concatenate/3  "wz"
  Constant7/1 -> MATLAB Function3/3(cutoff_freq), MATLAB Function1/3(cutoff_freq), MATLAB Function2/3(cutoff_freq)
  Demux/3 -> MATLAB Function3/1(curr_input)
  Constant6/1 -> MATLAB Function3/2(sample_freq)
  Demux/2 -> MATLAB Function1/1(curr_input)
  Demux/1 -> MATLAB Function2/1(curr_input), Scope/2
  gyro_B_rad/s_ori/1 -> Demux/1
  Constant2/1 -> MATLAB Function1/2(sample_freq)
  Constant4/1 -> MATLAB Function2/2(sample_freq)
  Vector Concatenate/1 -> gyro_B_rad/s_LPF/1

== system VB_RIFKF_UWB_INS25/No.1_Sensor_Data_Process1/Magn_Data_Process/Magn_preprocessing ==
  note: front-right-dowm
  Magn_B_rad/s_ori : Inport
  Constant2 : Constant  Value=1/dt  OutDataTypeStr=single
  Constant4 : Constant  Value=1/dt  OutDataTypeStr=single
  Constant6 : Constant  Value=1/dt  OutDataTypeStr=single
  Constant7 : Constant  Value=param.proces.imu_gyro_cutoff_freq  OutDataTypeStr=single
  Demux : Demux  Outputs=3
  MATLAB Function1 : MATLAB Function  TreatAsAtomicUnit=on
  MATLAB Function2 : MATLAB Function  TreatAsAtomicUnit=on
  MATLAB Function3 : MATLAB Function  TreatAsAtomicUnit=on
  Scope : Scope  NumInputPorts=2
  Vector Concatenate : Concatenate  NumInputs=3
  Magn_B_rad/s_LPF : Outport
  wires:
  Vector Concatenate/1 -> Magn_B_rad/s_LPF/1
  Constant4/1 -> MATLAB Function2/2(sample_freq)
  Constant2/1 -> MATLAB Function1/2(sample_freq)
  Magn_B_rad/s_ori/1 -> Demux/1
  Demux/1 -> Scope/2, MATLAB Function2/1(curr_input)
  Demux/2 -> MATLAB Function1/1(curr_input)
  Constant6/1 -> MATLAB Function3/2(sample_freq)
  Demux/3 -> MATLAB Function3/1(curr_input)
  Constant7/1 -> MATLAB Function2/3(cutoff_freq), MATLAB Function1/3(cutoff_freq), MATLAB Function3/3(cutoff_freq)
  MATLAB Function3/1(curr_output) -> Vector Concatenate/3  "wz"
  MATLAB Function1/1(curr_output) -> Vector Concatenate/2  "wy"
  MATLAB Function2/1(curr_output) -> Vector Concatenate/1  "wx"

== system VB_RIFKF_UWB_INS25/No.1_Sensor_Data_Process1/Subsystem/TD_baro ==
  H_baro : Inport
  Constant1 : Constant  Value=dt  OutDataTypeStr=single
  Constant3 : Constant  Value=0.1  OutDataTypeStr=single
  Constant4 : Constant  Value=900  OutDataTypeStr=single
  Delay1 : Delay  DelayLength=1  InitialConditionSource=Input port
      settings: InputPortMap=u0,p4
  MATLAB Function2 : MATLAB Function  TreatAsAtomicUnit=on
  Memory : Memory  InheritSampleTime=on
  Scope : Scope  NumInputPorts=3
  vH_baro_TD : Outport
  H_baro_TD : Outport  Port=2
  wires:
  Delay1/1 -> H_baro_TD/1, Scope/3, MATLAB Function2/3("u1 ")
  H_baro/1 -> Delay1/2, MATLAB Function2/2(u0), Scope/1
  Memory/1 -> MATLAB Function2/4("u2 "), vH_baro_TD/1, Scope/2
  Constant3/1 -> MATLAB Function2/5(h)
  Constant1/1 -> MATLAB Function2/1(T)
  Constant4/1 -> MATLAB Function2/6(r)
  MATLAB Function2/1(u1) -> Delay1/1
  MATLAB Function2/2(u2) -> Memory/1

== system VB_RIFKF_UWB_INS25/No.1_Sensor_Data_Process1/TOF_Data_Process/TD_baro ==
  H_TOF : Inport
  Constant1 : Constant  Value=dt  OutDataTypeStr=single
  Constant3 : Constant  Value=0.04  OutDataTypeStr=single
  Constant4 : Constant  Value=600  OutDataTypeStr=single
  Delay1 : Delay  DelayLength=1  InitialConditionSource=Input port
      settings: InputPortMap=u0,p4
  MATLAB Function2 : MATLAB Function  TreatAsAtomicUnit=on
  Memory : Memory  InheritSampleTime=on
  Scope : Scope  NumInputPorts=3
  vH_TOF_TD : Outport
  H_TOF_TD : Outport  Port=2
  wires:
  Delay1/1 -> H_TOF_TD/1, Scope/3, MATLAB Function2/3("u1 ")
  H_TOF/1 -> Delay1/2, MATLAB Function2/2(u0), Scope/1
  Memory/1 -> MATLAB Function2/4("u2 "), vH_TOF_TD/1, Scope/2
  Constant3/1 -> MATLAB Function2/5(h)
  Constant1/1 -> MATLAB Function2/1(T)
  Constant4/1 -> MATLAB Function2/6(r)
  MATLAB Function2/1(u1) -> Delay1/1
  MATLAB Function2/2(u2) -> Memory/1

== system VB_RIFKF_UWB_INS25/No.1_Sensor_Data_Process1/TOF_Data_Process/reinit_TOF ==
  QGC_sensor_reinit : Inport
  Data : Inport  Port=2
  Detect Increase : simulink/Logic and Bit Operations/Detect Increase  vinit=0.0  OutDataTypeStr=boolean
  Switch : Switch  Criteria=u2 > Threshold  SaturateOnIntegerOverflow=off  InputSameDT=off
  Unit Delay : UnitDelay  SampleTime=-1  HasFrameUpgradeWarning=on
  dataout : Outport
  wires:
  Unit Delay/1 -> Switch/3
  Data/1 -> Switch/1
  Switch/1 -> dataout/1, Unit Delay/1
  Detect Increase/1 -> Switch/2
  QGC_sensor_reinit/1 -> Detect Increase/1

== system VB_RIFKF_UWB_INS25/No.1_Sensor_Data_Process1/baro_Data_Process/Pressure2Height ==
  baro : Inport
  Add : Sum  Inputs=+-
  Constant : Constant  OutDataTypeStr=single
  Constant1 : Constant  Value=1/5.255  OutDataTypeStr=single
  Gain : Gain  Gain=1/1.01325
  Gain1 : Gain  Gain=44330
  Math Function : Math  Operator=pow  SignedPower=on
  H_baro : Outport
  wires:
  Gain/1 -> Math Function/1
  Constant1/1 -> Math Function/2
  Math Function/1 -> Add/2
  Constant/1 -> Add/1
  Add/1 -> Gain1/1
  Gain1/1 -> H_baro/1
  baro/1 -> Gain/1

== system VB_RIFKF_UWB_INS25/No.1_Sensor_Data_Process1/baro_Data_Process/TD_baro ==
  H_baro : Inport
  Constant1 : Constant  Value=dt  OutDataTypeStr=single
  Constant3 : Constant  Value=0.23  OutDataTypeStr=single
  Constant4 : Constant  Value=900  OutDataTypeStr=single
  Delay1 : Delay  DelayLength=1  InitialConditionSource=Input port
      settings: InputPortMap=u0,p4
  MATLAB Function2 : MATLAB Function  TreatAsAtomicUnit=on
  Memory : Memory  InheritSampleTime=on
  Scope : Scope  NumInputPorts=3
  vH_baro_TD : Outport
  H_baro_TD : Outport  Port=2
  wires:
  Delay1/1 -> H_baro_TD/1, Scope/3, MATLAB Function2/3("u1 ")
  H_baro/1 -> Delay1/2, MATLAB Function2/2(u0), Scope/1
  Memory/1 -> MATLAB Function2/4("u2 "), vH_baro_TD/1, Scope/2
  Constant3/1 -> MATLAB Function2/5(h)
  Constant1/1 -> MATLAB Function2/1(T)
  Constant4/1 -> MATLAB Function2/6(r)
  MATLAB Function2/1(u1) -> Delay1/1
  MATLAB Function2/2(u2) -> Memory/1

== system VB_RIFKF_UWB_INS25/No.1_Sensor_Data_Process1/baro_Data_Process/TemCompensate1 ==
  baro_tem : Inport
  Add : Sum  Inputs=+++
  Constant2 : Constant  Value=-1663  OutDataTypeStr=single
  Gain : Gain  Gain=-1.6
  Gain1 : Gain  Gain=102.5
  Product : Product
  bias : Outport
  wires:
  Gain1/1 -> Add/2
  Add/1 -> bias/1
  Gain/1 -> Add/1
  Product/1 -> Gain/1
  Constant2/1 -> Add/3
  baro_tem/1 -> Product/1, Product/2, Gain1/1

== system VB_RIFKF_UWB_INS25/No.1_Sensor_Data_Process1/baro_Data_Process/reinit_baro0 ==
  QGC_sensor_reinit : Inport
  Data : Inport  Port=2
  Detect Increase : simulink/Logic and Bit Operations/Detect Increase  vinit=0.0  OutDataTypeStr=boolean
  Switch : Switch  Criteria=u2 > Threshold  SaturateOnIntegerOverflow=off  InputSameDT=off
  Unit Delay : UnitDelay  SampleTime=-1  HasFrameUpgradeWarning=on
  dataout : Outport
  wires:
  Unit Delay/1 -> Switch/3
  Data/1 -> Switch/1
  Switch/1 -> dataout/1, Unit Delay/1
  Detect Increase/1 -> Switch/2
  QGC_sensor_reinit/1 -> Detect Increase/1

== system VB_RIFKF_UWB_INS25/No.1_Sensor_Data_Process1/baro_Data_Process/reinit_baro1 ==
  QGC_sensor_reinit : Inport
  Data : Inport  Port=2
  Detect Increase : simulink/Logic and Bit Operations/Detect Increase  vinit=0.0  OutDataTypeStr=boolean
  Switch : Switch  Criteria=u2 > Threshold  SaturateOnIntegerOverflow=off  InputSameDT=off
  Unit Delay : UnitDelay  SampleTime=-1  HasFrameUpgradeWarning=on
  dataout : Outport
  wires:
  QGC_sensor_reinit/1 -> Detect Increase/1
  Detect Increase/1 -> Switch/2
  Switch/1 -> Unit Delay/1, dataout/1
  Data/1 -> Switch/1
  Unit Delay/1 -> Switch/3

== system VB_RIFKF_UWB_INS25/No.1_Sensor_Data_Process2/GPS_Data_Process/LLA2NED ==
  note: Vecef2ned
  gps_LLA_rad : Inport
  GPSfixtype : Inport  Port=2
  GPS_Vecef_m/s : Inport  Port=3
  QGC_sensor_reinit : Inport  Port=4
  GPS0 : Inport  Port=5
  Angle Conversion1 : aerolibconvert2/Angle Conversion  IU=deg  OU=rad
  Bus Creator : BusCreator  Inputs=3
  Bus Creator1 : BusCreator  Inputs=3
  Bus Selector : BusSelector  OutputSignals=lon_gps,lat_gps
  Bus Selector1 : BusSelector  OutputSignals=lat_gps,lon_gps,H_gps
  Constant1 : Constant  Value=-90
  Constant4 : Constant  Value=0
  Data Type Conversion{,1..3} (4 alike) : DataTypeConversion  OutDataTypeStr=single  SaturateOnIntegerOverflow=off  RndMeth=Floor
  Demux : Demux  Outputs=3
  Demux1 : Demux  Outputs=3
  Demux3 : Demux  Outputs=3
  Detect Increase : simulink/Logic and Bit Operations/Detect Increase  vinit=0.0  OutDataTypeStr=boolean
  Direction Cosine Matrix ECEF to NED : aerolibtransform2/Direction Cosine Matrix ECEF to NED  Commented=on
  Divide1 : Product  Inputs=**  Multiplication=Matrix(*)
  Gain : Gain  Gain=-1
  LLA to ECEF Position : LLA2ECEF  R=6378137
  LLA to ECEF Position1 : LLA2ECEF  R=6378137
  Mux2 : Mux  Inputs=3
  Mux5 : Mux  Inputs=2
  Mux6 : Mux  Inputs=2
  Product : Product  Commented=on  Multiplication=Matrix(*)
  Radians to Degrees{,1..3} (4 alike) : simulink_extras/Transformations/Radians to Degrees
  Radians to Degrees4 : simulink_extras/Transformations/Radians to Degrees  Commented=on
  Rotation Angles to Direction Cosine Matrix : sharedtransform/Rotation Angles to Direction Cosine Matrix  rotationOrder=ZYX  aMode=aMode
  Scope1 : Scope
  Selector2 : Selector  Commented=on  InputPortWidth=3  IndexOptions=Index vector (dialog)  Indices=[1 2]  OutputSizes=1
  Sum : Sum  Inputs=|++
  Sum1 : Sum  Inputs=|+-
  initGPSLLA : MATLAB Function  TreatAsAtomicUnit=on
  "gpsposNEDout " : Outport
  gpsvNEDout : Outport  Port=2
  wires:
  initGPSLLA/1(gpsLLA0_rad) -> Demux/1
  Detect Increase/1 -> initGPSLLA/1(QGCinitflag)
  Data Type Conversion3/1 -> gpsvNEDout/1  "gpspos_N"
  Radians to Degrees4/1 -> Direction Cosine Matrix ECEF to NED/1
  Selector2/1 -> Radians to Degrees4/1
  Direction Cosine Matrix ECEF to NED/1 -> Product/1
  GPS_Vecef_m/s/1 -> Product/2, Data Type Conversion3/1
  Radians to Degrees3/1 -> Mux5/2
  Radians to Degrees2/1 -> Mux5/1
  Angle Conversion1/1 -> Sum/2
  Data Type Conversion2/1 -> Bus Creator1/3  "gpspos_D"
  Data Type Conversion1/1 -> Bus Creator1/2  "gpspos_E"
  Data Type Conversion/1 -> Bus Creator1/1  "gpspos_N"
  QGC_sensor_reinit/1 -> Detect Increase/1
  Radians to Degrees1/1 -> Mux6/2
  Radians to Degrees/1 -> Mux6/1
  gps_LLA_rad/1 -> Demux1/1, Selector2/1, initGPSLLA/3(gps_LLA_rad)
  Bus Selector1/3 -> LLA to ECEF Position/2  "<H_gps>"
  Bus Selector1/2 -> Radians to Degrees3/1  "<lon_gps>"
  Bus Selector1/1 -> Radians to Degrees2/1  "<lat_gps>"
  Bus Selector/1 -> Mux2/1  "<lon_gps>"
  Bus Selector/2 -> Gain/1  "<lat_gps>"
  Sum/1 -> Mux2/2
  Demux1/2 -> Radians to Degrees1/1
  LLA to ECEF Position/1 -> Sum1/2
  Constant1/1 -> Angle Conversion1/1
  Rotation Angles to Direction Cosine Matrix/1 -> Divide1/1
  Mux2/1 -> Rotation Angles to Direction Cosine Matrix/1
  Demux1/1 -> Radians to Degrees/1
  Divide1/1 -> Demux3/1
  Sum1/1 -> Divide1/2
  Constant4/1 -> Mux2/3
  LLA to ECEF Position1/1 -> Sum1/1
  Gain/1 -> Sum/1
  Mux5/1 -> LLA to ECEF Position/1
  Mux6/1 -> LLA to ECEF Position1/1
  Demux1/3 -> LLA to ECEF Position1/2
  Demux/1 -> Bus Creator/1  "lat_gps"
  Demux/2 -> Bus Creator/2  "lon_gps"
  Demux/3 -> Bus Creator/3  "H_gps"
  Bus Creator/1 -> Bus Selector/1, Bus Selector1/1
  Demux3/1 -> Data Type Conversion/1  "gpspos_N"
  Demux3/2 -> Data Type Conversion1/1  "gpspos_E"
  Demux3/3 -> Data Type Conversion2/1  "gpspos_D"
  Bus Creator1/1 -> Scope1/1, "gpsposNEDout "/1
  GPSfixtype/1 -> initGPSLLA/2(GPSfixtype)

== system VB_RIFKF_UWB_INS25/No.1_Sensor_Data_Process2/GPS_Data_Process/heading_GPS ==
  Vned : Inport
  Atan2 : Trigonometry  Operator=atan2
  Compare To Constant : simulink/Logic and Bit Operations/Compare To Constant  relop=>=  const=0.8  OutDataTypeStr=boolean
  Math Function : Math  Operator=magnitude^2  SignedPower=on
  Moving Average1 : dspstat3/Moving Average  Commented=on  Method=Sliding window  ForgettingFactorPort=off  SpecifyWindowLength=on  WindowLength=10  OverlapLength=9  AllowArbitraryInputLength=off  ForgettingFactor=0.9  SimulateUsing=Code generation
  Scope : Scope  NumInputPorts=2
  Scope1 : Scope
  Selector2 : Selector  InputPortWidth=3  IndexOptions=Index vector (dialog)  Indices=[2]  OutputSizes=1
  Selector3 : Selector  InputPortWidth=3  IndexOptions=Index vector (dialog)  Indices=[1]  OutputSizes=1
  Selector4 : Selector  InputPortWidth=3  IndexOptions=Index vector (dialog)  Indices=[1 2]  OutputSizes=1
  Sqrt : Sqrt
  Sum of Elements : Sum  Inputs=+
  heading_GPS_rad : Outport
  heading_GPS_valid : Outport  Port=2
  wires:
  Atan2/1 -> heading_GPS_rad/1, Scope/2, Scope/1
  Compare To Constant/1 -> heading_GPS_valid/1, Scope1/1
  Sqrt/1 -> Compare To Constant/1
  Selector4/1 -> Math Function/1
  Sum of Elements/1 -> Sqrt/1
  Selector3/1 -> Atan2/2
  Vned/1 -> Selector3/1, Selector4/1, Selector2/1
  Math Function/1 -> Sum of Elements/1
  Selector2/1 -> Atan2/1
